simulink model "VehicleFollowing_R2019a"  (R2019a)
settings: Solver=VariableStepAuto  StartTime=0.0  StopTime=50  RelTol=1e-3
libraries: simulink x3, sim3dautolib x3, vrlib x2, sim3dlib x1, mpcadaslib x1, robotmobilelib x1
settings Model: Creator=Mustafa  LastModifiedBy=mustafa

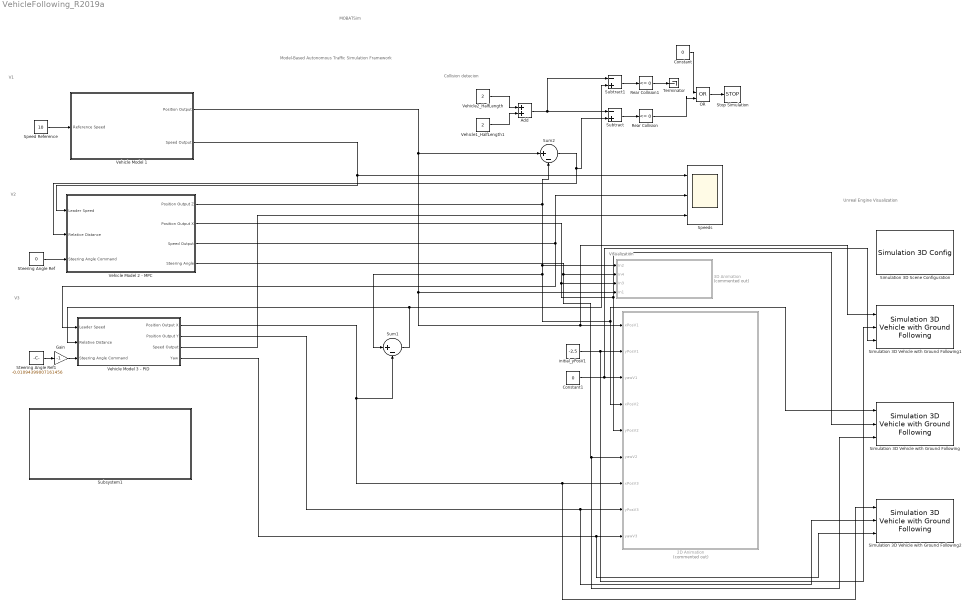
== system VehicleFollowing_R2019a ==
  note: Unreal Engine Visualization
  note: V1
  note: Visualization
  note: Collision detecion
  note: Model-Based Autonomous Traffic Simulation Framework
  note: MOBATSim
  note: V2
  note: V3
  2D Animation : Subsystem  Commented=on  TreatAsAtomicUnit=on  SystemSampleTime=0.02
  3D Animation : Subsystem  Commented=on
  Add : Sum
  Constant : Constant  Value=0
  Constant1 : Constant  Value=0
  Gain : Gain  Gain=-1
  OR : Logic  Operator=OR  IconShape=distinctive  AllPortsSameDT=off  OutDataTypeStr=boolean
  Rear Collision : simulink/Logic and Bit Operations/Compare To Constant  relop=<=  const=0  OutDataTypeStr=boolean
  Rear Collision1 : simulink/Logic and Bit Operations/Compare To Constant  relop=<=  const=0  OutDataTypeStr=boolean
  Simulation 3D Scene Configuration : sim3dlib/Simulation 3D Config  Priority=0  ProjectFormat=Default Scenes  SceneDesc=Straight road  ProjectName=VehicleSimulation.exe  vehTagList={'Scene Origin';'SimulinkVehicle1';'SimulinkVehicle2';'SimulinkVehicle3'}  vehTag=SimulinkVehicle3  OpVisEn=off  Ts=0.1  aMode=3
      settings: SourceProductBaseCode=DR,UV,VE
  Simulation 3D Vehicle with Ground Following : sim3dautolib/Simulation 3D Vehicle with Ground Following  Priority=-1  PassVehMesh=Small pickup truck  VehColor=Orange  InitialPos=[20, 0, 0]  InitialRot=[0, 0, 0]  ActorName=SimulinkVehicle1  SampleTime=0.1  ActorType=SimulinkVehicle  ID=1  aMode=3  ActorTag=SimulinkVehicle1  CoordinateScheme=ISO  TransformOutportEnabled=off
      settings: SourceProductBaseCode=DR,UV,VE
  Simulation 3D Vehicle with Ground Following1 : sim3dautolib/Simulation 3D Vehicle with Ground Following  Priority=-1  PassVehMesh=Muscle car  VehColor=Red  InitialPos=[40, 0, 0]  InitialRot=[0, 0, 0]  ActorName=SimulinkVehicle2  SampleTime=0.1  ActorType=SimulinkVehicle  ID=2  aMode=3  ActorTag=SimulinkVehicle2  CoordinateScheme=ISO  TransformOutportEnabled=off
      settings: SourceProductBaseCode=DR,UV,VE
  Simulation 3D Vehicle with Ground Following2 : sim3dautolib/Simulation 3D Vehicle with Ground Following  Priority=-1  PassVehMesh=Sedan  VehColor=Silver  InitialPos=[0, 0, 0]  InitialRot=[0, 0, 0]  ActorName=SimulinkVehicle3  SampleTime=0.1  ActorType=SimulinkVehicle  ID=3  aMode=3  ActorTag=SimulinkVehicle3  CoordinateScheme=ISO  TransformOutportEnabled=off
      settings: SourceProductBaseCode=DR,UV,VE
  Speed Reference : Constant  Value=10
  Speeds : Scope  NumInputPorts=3
  Steering Angle Ref : Constant  Value=0
  Steering Angle Ref1 : Constant  Value=-0.01094399007161456
  Stop Simulation : Stop
  Subsystem1 : Subsystem
  Subtract : Sum  Inputs=-+
  Subtract1 : Sum  Inputs=-+
  Sum1 : Sum  Inputs=|+-
  Sum2 : Sum  Inputs=|+-
  Terminator : Terminator
  Vehicle Model 1 : Subsystem  mask{Pos=40, Speed=20}
      mask prompts: Pos "Initial Position"; Speed "Initial Speed"
      mask TypeOptions Pos: Initial Position/Value
      mask TypeOptions Speed: Initial Speed/Value
  Vehicle Model 2 - MPC : Subsystem  mask{Pos=20, Speed=25}
      mask prompts: Pos "Initial Position"; Speed "Initial Speed"
      mask TypeOptions Pos: Initial Position Z/Value
      mask TypeOptions Speed: Initial Speed/Value
  Vehicle Model 3 - PID : Subsystem  mask{Pos=0, Speed=10}
      mask prompts: Pos "Initial Position"; Speed "Initial Speed"
      mask TypeOptions Pos: Initial Position X/Value
      mask TypeOptions Speed: Initial Speed/Value
  Vehicle1_HalfLength1 : Constant  Value=2
  Vehicle2_HalfLength : Constant  Value=2
  initial_yPosV1 : Constant  Value=-2.5
  wires:
  Vehicle Model 2 - MPC/1(Position Output Z) -> Sum1/1, 2D Animation/4(xPosV2), Simulation 3D Vehicle with Ground Following/1, 3D Animation/1(In2), Sum2/2
  Vehicle Model 2 - MPC/3(Speed Output) -> Vehicle Model 3 - PID/1(Leader Speed), Speeds/2
  Speed Reference/1 -> Vehicle Model 1/1(Reference Speed)
  Vehicle Model 1/1(Position Output) -> Sum2/1, Simulation 3D Vehicle with Ground Following1/1, 2D Animation/1(xPosV1), 3D Animation/4(In1)
  Sum2/1 -> Subtract/2, Vehicle Model 2 - MPC/2(Relative Distance)
  Vehicle Model 1/2(Speed Output) -> Vehicle Model 2 - MPC/1(Leader Speed), Speeds/1
  Steering Angle Ref/1 -> Vehicle Model 2 - MPC/3(Steering Angle Command)
  Vehicle Model 2 - MPC/2(Position Output X) -> 2D Animation/5(yPosV2), Simulation 3D Vehicle with Ground Following/2, 3D Animation/3(In3)
  Vehicle Model 2 - MPC/4(Steering Angle) -> Simulation 3D Vehicle with Ground Following/3, 2D Animation/6(yawV2), 3D Animation/2(In4)
  initial_yPosV1/1 -> Simulation 3D Vehicle with Ground Following1/2, 2D Animation/2(yPosV1)
  Constant1/1 -> Simulation 3D Vehicle with Ground Following1/3, 2D Animation/3(yawV1)
  Vehicle1_HalfLength1/1 -> Add/2
  Vehicle2_HalfLength/1 -> Add/1
  Add/1 -> Subtract1/1, Subtract/1
  Subtract/1 -> Rear Collision/1
  Vehicle Model 3 - PID/1(Position Output X) -> Simulation 3D Vehicle with Ground Following2/1, 2D Animation/7(xPosV3), Sum1/2
  Vehicle Model 3 - PID/2(Position Output Y) -> Simulation 3D Vehicle with Ground Following2/2, 2D Animation/8(yPosV3)
  Vehicle Model 3 - PID/3(Speed Output) -> Speeds/3
  Vehicle Model 3 - PID/4(Yaw) -> Simulation 3D Vehicle with Ground Following2/3, 2D Animation/9(yawV3)
  Sum1/1 -> Vehicle Model 3 - PID/2(Relative Distance), Subtract1/2
  OR/1 -> Stop Simulation/1
  Rear Collision/1 -> OR/2
  Subtract1/1 -> Rear Collision1/1
  Steering Angle Ref1/1 -> Gain/1
  Constant/1 -> OR/1
  Rear Collision1/1 -> Terminator/1
  Gain/1 -> Vehicle Model 3 - PID/3(Steering Angle Command)

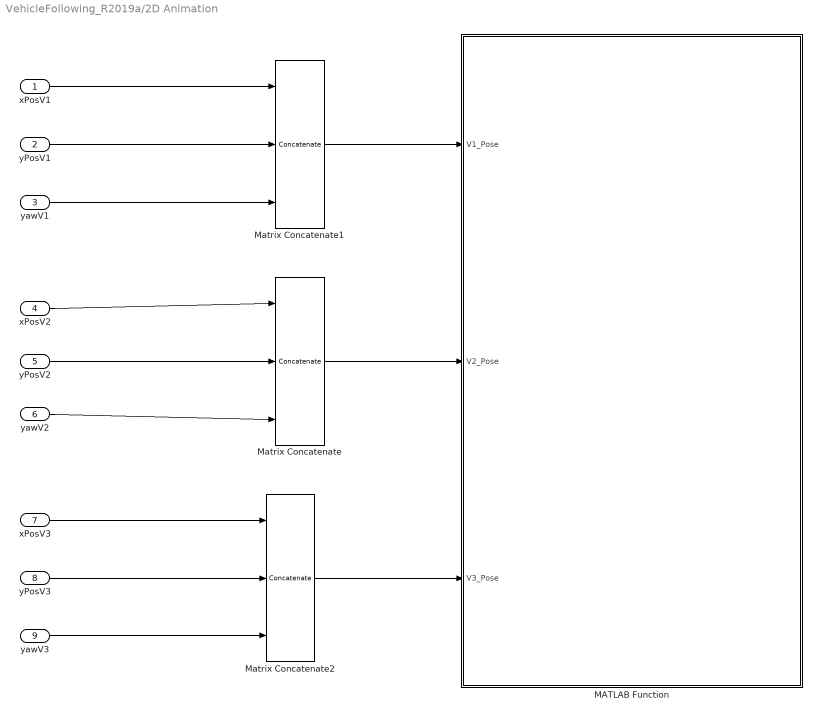
== system VehicleFollowing_R2019a/2D Animation ==
  xPosV1 : Inport
  yPosV1 : Inport  Port=2
  yawV1 : Inport  Port=3
  xPosV2 : Inport  Port=4
  yPosV2 : Inport  Port=5
  yawV2 : Inport  Port=6
  xPosV3 : Inport  Port=7
  yPosV3 : Inport  Port=8
  yawV3 : Inport  Port=9
  MATLAB Function : MATLAB Function  TreatAsAtomicUnit=on
      mask init:
      | close all;
      | figure('units','normalized','outerposition',[0 0 1 1]);
      | grid on
      | axis equal
      | hold on
  Matrix Concatenate : Concatenate  NumInputs=3  ConcatenateDimension=2
  Matrix Concatenate1 : Concatenate  NumInputs=3  ConcatenateDimension=2
  Matrix Concatenate2 : Concatenate  NumInputs=3  ConcatenateDimension=2
  wires:
  xPosV2/1 -> Matrix Concatenate/1
  Matrix Concatenate/1 -> MATLAB Function/2(V2_Pose)
  yPosV2/1 -> Matrix Concatenate/2
  yawV2/1 -> Matrix Concatenate/3
  Matrix Concatenate1/1 -> MATLAB Function/1(V1_Pose)
  xPosV1/1 -> Matrix Concatenate1/1
  yPosV1/1 -> Matrix Concatenate1/2
  yawV1/1 -> Matrix Concatenate1/3
  yPosV3/1 -> Matrix Concatenate2/2
  xPosV3/1 -> Matrix Concatenate2/1
  yawV3/1 -> Matrix Concatenate2/3
  Matrix Concatenate2/1 -> MATLAB Function/3(V3_Pose)

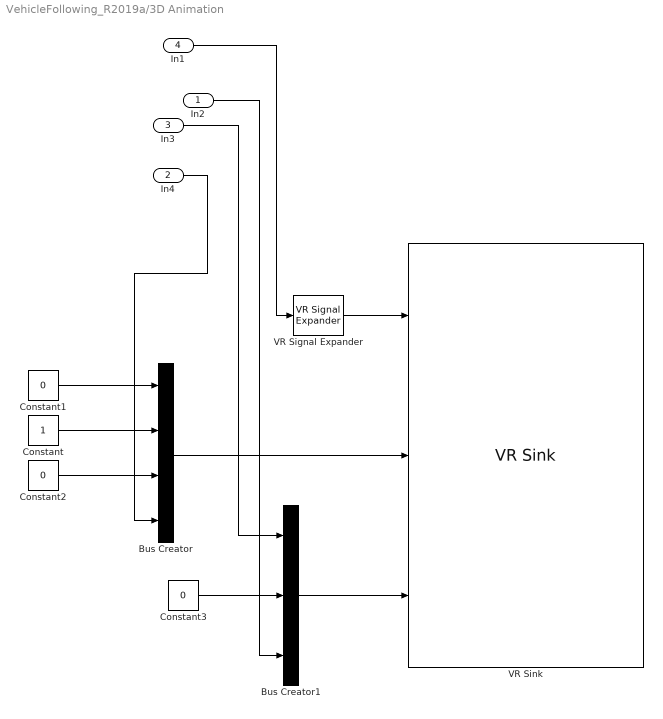
== system VehicleFollowing_R2019a/3D Animation ==
  In2 : Inport
  In4 : Inport  Port=2
  In3 : Inport  Port=3
  In1 : Inport  Port=4
  Bus Creator : BusCreator  Inputs=4
  Bus Creator1 : BusCreator  Inputs=3
  Constant : Constant
  Constant1 : Constant  Value=0
  Constant2 : Constant  Value=0
  Constant3 : Constant  Value=0
  VR Signal Expander : vrlib/VR Signal Expander  outwidth=3  outidx=[3]
  VR Sink : vrlib/VR Sink  InstantiateOnLoad=on  SampleTime=0.02  ViewEnable=on  RemoteChange=off  RemoteView=off  FieldsWritten=Car_Red.translation.3.1.1.double#Car_Blue.rotation.4.1.1.double#Car_Blue.translation.3.1.1.double  WorldFileName=PlatoonWorld.WRL  AutoView=off  VideoDimensions=[]  AllowVariableSize=off
  wires:
  Constant/1 -> Bus Creator/2
  Constant1/1 -> Bus Creator/1
  Bus Creator1/1 -> VR Sink/3
  In2/1 -> Bus Creator1/3
  Bus Creator/1 -> VR Sink/2
  In4/1 -> Bus Creator/4
  In1/1 -> VR Signal Expander/1
  Constant3/1 -> Bus Creator1/2
  Constant2/1 -> Bus Creator/3
  VR Signal Expander/1 -> VR Sink/1
  In3/1 -> Bus Creator1/1

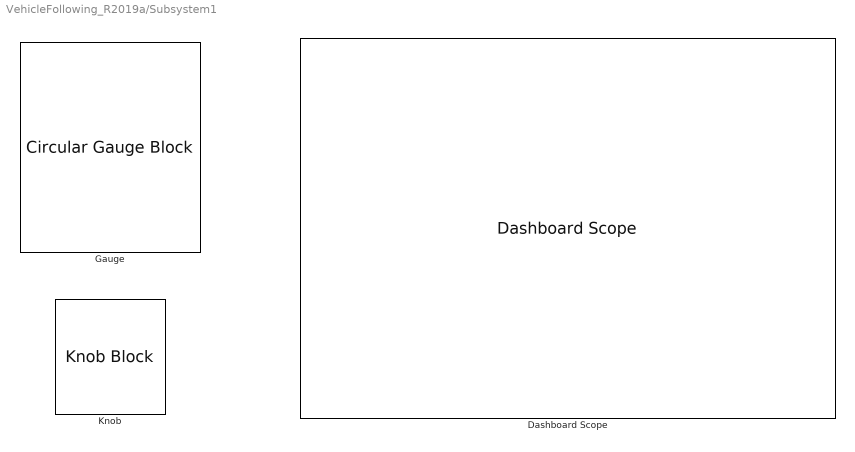
== system VehicleFollowing_R2019a/Subsystem1 ==
  Dashboard Scope : DashboardScope  WebBlockId=244
  Gauge : CircularGaugeBlock  WebBlockId=245
  Knob : KnobBlock  ScaleMin=-0.2  ScaleMax=0.2  WebBlockId=247

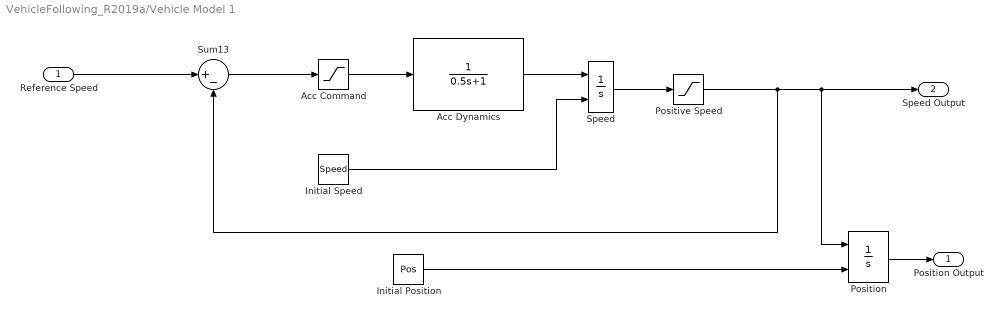
== system VehicleFollowing_R2019a/Vehicle Model 1 ==
  Reference Speed : Inport
  Acc Command : Saturate  UpperLimit=2  LowerLimit=-3
  Acc Dynamics : TransferFcn  Denominator=[0.5 1]
  Initial Position : Constant  Value=Pos
  Initial Speed : Constant  Value=Speed
  Position : Integrator  InitialConditionSource=external
  Positive Speed : Saturate  UpperLimit=inf  LowerLimit=0
  Speed : Integrator  InitialConditionSource=external
  Sum13 : Sum  Inputs=|+-
  Position Output : Outport  VectorParamsAs1DForOutWhenUnconnected=off
  Speed Output : Outport  Port=2  VectorParamsAs1DForOutWhenUnconnected=off
  wires:
  Speed/1 -> Positive Speed/1
  Positive Speed/1 -> Sum13/2, Speed Output/1, Position/1
  Initial Position/1 -> Position/2
  Sum13/1 -> Acc Command/1
  Reference Speed/1 -> Sum13/1
  Acc Command/1 -> Acc Dynamics/1
  Acc Dynamics/1 -> Speed/1
  Initial Speed/1 -> Speed/2
  Position/1 -> Position Output/1

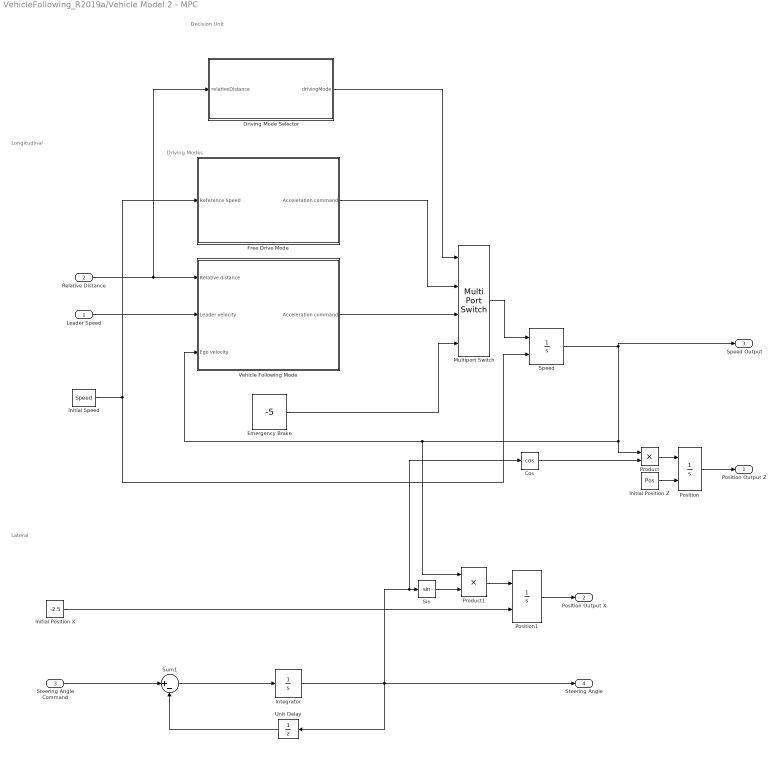
== system VehicleFollowing_R2019a/Vehicle Model 2 - MPC ==
  note: Decision Unit
  note: Driving Modes
  note: Longitudinal
  note: Lateral
  Leader Speed : Inport
  Relative Distance : Inport  Port=2
  Steering Angle Command : Inport  Port=3
  Cos : Trigonometry  Operator=cos
  Driving Mode Selector : Stateflow chart  TreatAsAtomicUnit=on
  Emergency Brake : Constant  Value=-5
  Free Drive Mode : Subsystem
  Initial Position X : Constant  Value=-2.5
  Initial Position Z : Constant  Value=Pos
  Initial Speed : Constant  Value=Speed
  Integrator : Integrator
  Multiport Switch : MultiPortSwitch
  Position : Integrator  InitialConditionSource=external
  Position1 : Integrator  InitialConditionSource=external
  Product : Product
  Product1 : Product
  Sin : Trigonometry
  Speed : Integrator  InitialConditionSource=external  LimitOutput=on  LowerSaturationLimit=0
  Sum1 : Sum  Inputs=|+-
  Unit Delay : UnitDelay  SampleTime=-1  HasFrameUpgradeWarning=on
  Vehicle Following Mode : Subsystem
  Position Output Z : Outport  VectorParamsAs1DForOutWhenUnconnected=off
  Position Output X : Outport  Port=2  VectorParamsAs1DForOutWhenUnconnected=off
  Speed Output : Outport  Port=3  VectorParamsAs1DForOutWhenUnconnected=off
  Steering Angle : Outport  Port=4  VectorParamsAs1DForOutWhenUnconnected=off
  wires:
  Position/1 -> Position Output Z/1
  Initial Speed/1 -> Free Drive Mode/1(Reference Speed), Speed/2
  Initial Position Z/1 -> Position/2
  Speed/1 -> Speed Output/1, Vehicle Following Mode/3(Ego velocity), Product1/1, Product/1
  Steering Angle Command/1 -> Sum1/1
  Sum1/1 -> Integrator/1
  Integrator/1 -> Unit Delay/1, Sin/1, Cos/1, Steering Angle/1
  Unit Delay/1 -> Sum1/2
  Initial Position X/1 -> Position1/2
  Cos/1 -> Product/2
  Product/1 -> Position/1
  Sin/1 -> Product1/2
  Product1/1 -> Position1/1
  Position1/1 -> Position Output X/1
  Relative Distance/1 -> Driving Mode Selector/1(relativeDistance), Vehicle Following Mode/1(Relative distance)
  Leader Speed/1 -> Vehicle Following Mode/2(Leader velocity)
  Vehicle Following Mode/1(Acceleration command) -> Multiport Switch/3
  Multiport Switch/1 -> Speed/1
  Free Drive Mode/1(Acceleration command) -> Multiport Switch/2
  Emergency Brake/1 -> Multiport Switch/4
  Driving Mode Selector/1(drivingMode) -> Multiport Switch/1

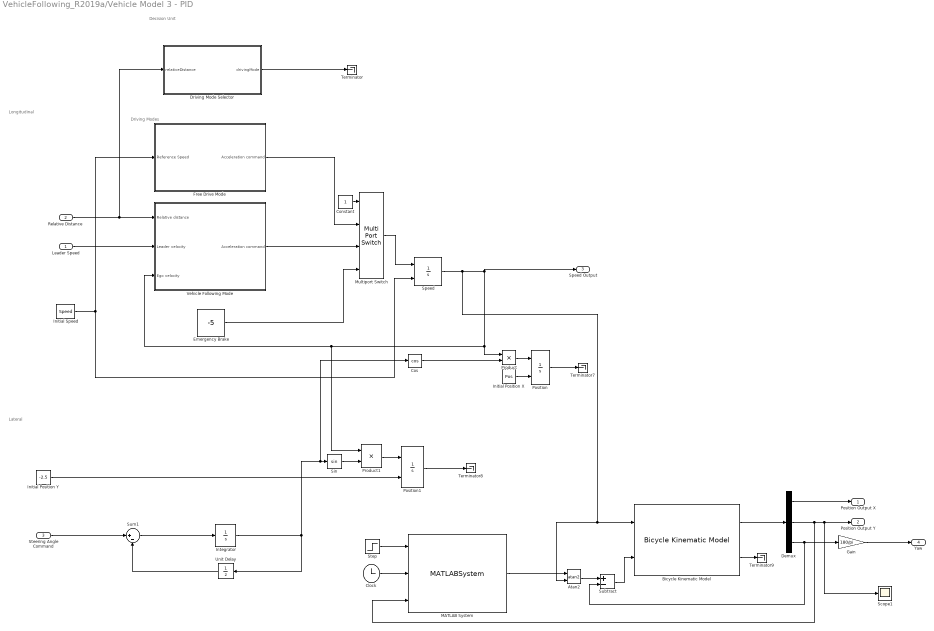
== system VehicleFollowing_R2019a/Vehicle Model 3 - PID ==
  note: Decision Unit
  note: Driving Modes
  note: Longitudinal
  note: Lateral
  Leader Speed : Inport
  Relative Distance : Inport  Port=2
  Steering Angle Command : Inport  Port=3
  Atan2 : Trigonometry  Operator=atan2
  Bicycle Kinematic Model : robotmobilelib/Bicycle Kinematic Model  VehicleInputs=Vehicle Speed & Steering Angle  WheelBase=3  VehicleSpeedRange=[0 12]  MaxSteeringAngle=pi/4  InitialState=[0; -3; 0]  SimulateUsing=Interpreted execution
      settings: SourceProductBaseCode=RO
  Clock : Clock
  Constant : Constant
  Cos : Trigonometry  Operator=cos
  Demux : Demux  Outputs=3
  Driving Mode Selector : Stateflow chart  TreatAsAtomicUnit=on
  Emergency Brake : Constant  Value=-5
  Free Drive Mode : Subsystem
  Gain : Gain  Gain=180/pi
  Initial Position X : Constant  Value=Pos
  Initial Position Y : Constant  Value=-2.5
  Initial Speed : Constant  Value=Speed
  Integrator : Integrator
  MATLAB System : MATLABSystem  System=LaneChanger  SimulateUsing=Interpreted execution
      mask Type: LaneChanger
      mask Display:
      | disp('LaneChanger');
      | port_label('input',1,'flag');
      | port_label('input',2,'clock');
      | port_label('input',3,'y');
      | port_label('output',1,'latSpeed');
  Multiport Switch : MultiPortSwitch
  Position : Integrator  InitialConditionSource=external
  Position1 : Integrator  InitialConditionSource=external
  Product : Product
  Product1 : Product
  Scope1 : Scope
  Sin : Trigonometry
  Speed : Integrator  InitialConditionSource=external  LimitOutput=on  UpperSaturationLimit=12  LowerSaturationLimit=0
  Step : Step  Time=3  SampleTime=0
  Subtract : Sum  Inputs=+-
  Sum1 : Sum  Inputs=|+-
  Terminator{,7..9} (4 alike) : Terminator
  Unit Delay : UnitDelay  SampleTime=-1  HasFrameUpgradeWarning=on
  Vehicle Following Mode : Subsystem
  Position Output X : Outport  VectorParamsAs1DForOutWhenUnconnected=off
  Position Output Y : Outport  Port=2  VectorParamsAs1DForOutWhenUnconnected=off
  Speed Output : Outport  Port=3  VectorParamsAs1DForOutWhenUnconnected=off
  Yaw : Outport  Port=4  VectorParamsAs1DForOutWhenUnconnected=off
  wires:
  Initial Speed/1 -> Free Drive Mode/1(Reference Speed), Speed/2
  Initial Position X/1 -> Position/2
  Speed/1 -> Atan2/2, Bicycle Kinematic Model/1, Speed Output/1, Vehicle Following Mode/3(Ego velocity), Product1/1, Product/1
  Sum1/1 -> Integrator/1
  Integrator/1 -> Unit Delay/1, Sin/1, Cos/1
  Unit Delay/1 -> Sum1/2
  Initial Position Y/1 -> Position1/2
  Cos/1 -> Product/2
  Product/1 -> Position/1
  Sin/1 -> Product1/2
  Product1/1 -> Position1/1
  Relative Distance/1 -> Driving Mode Selector/1(relativeDistance), Vehicle Following Mode/1(Relative distance)
  Leader Speed/1 -> Vehicle Following Mode/2(Leader velocity)
  Vehicle Following Mode/1(Acceleration command) -> Multiport Switch/3
  Multiport Switch/1 -> Speed/1
  Free Drive Mode/1(Acceleration command) -> Multiport Switch/2
  Emergency Brake/1 -> Multiport Switch/4
  Driving Mode Selector/1(drivingMode) -> Terminator/1
  Constant/1 -> Multiport Switch/1
  Position/1 -> Terminator7/1
  Position1/1 -> Terminator8/1
  Gain/1 -> Yaw/1
  Bicycle Kinematic Model/1 -> Demux/1
  Bicycle Kinematic Model/2 -> Terminator9/1
  Demux/3 -> Subtract/2, Gain/1
  Demux/2 -> MATLAB System/3, Scope1/1, Position Output Y/1
  Demux/1 -> Position Output X/1
  Steering Angle Command/1 -> Sum1/1
  Step/1 -> MATLAB System/1
  Clock/1 -> MATLAB System/2
  MATLAB System/1 -> Atan2/1
  Atan2/1 -> Subtract/1
  Subtract/1 -> Bicycle Kinematic Model/2

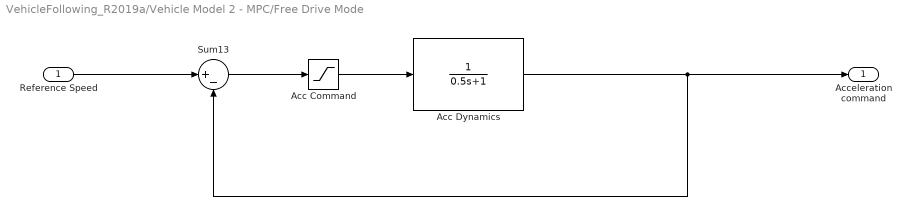
== system VehicleFollowing_R2019a/Vehicle Model 2 - MPC/Free Drive Mode ==
  Reference Speed : Inport
  Acc Command : Saturate  UpperLimit=2  LowerLimit=-3
  Acc Dynamics : TransferFcn  Denominator=[0.5 1]
  Sum13 : Sum  Inputs=|+-
  Acceleration command : Outport
  wires:
  Sum13/1 -> Acc Command/1
  Acc Dynamics/1 -> Acceleration command/1, Sum13/2
  Reference Speed/1 -> Sum13/1
  Acc Command/1 -> Acc Dynamics/1

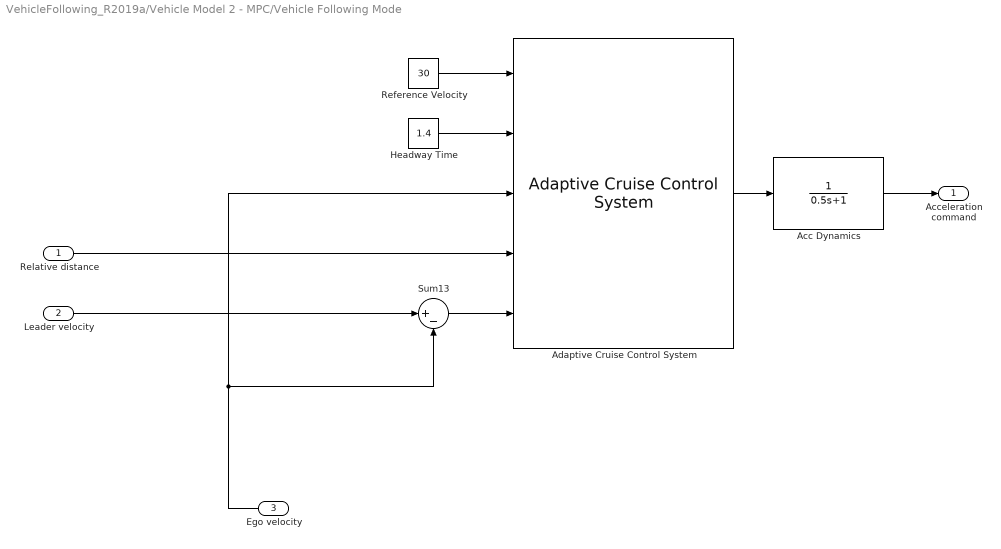
== system VehicleFollowing_R2019a/Vehicle Model 2 - MPC/Vehicle Following Mode ==
  Relative distance : Inport
  Leader velocity : Inport  Port=2
  Ego velocity : Inport  Port=3
  Acc Dynamics : TransferFcn  Denominator=[0.5 1]
  Adaptive Cruise Control System : mpcadaslib/Adaptive Cruise Control System  EgoModel=tf(1,[0.5,1,0])  InitialEgoVelocity=30  DefaultSpacing=10  MaxVelocity=50  MinAcceleration=-3  amin_ext=off  MaxAcceleration=2  amax_ext=off  Ts=0.5  PredictionHorizon=200  ControllerBehavior=0.590  suboptimal=off  maxiter=100  datatypeopt=double  optmode=off  trackmode=off
  Headway Time : Constant  Value=1.4
  Reference Velocity : Constant  Value=30
  Sum13 : Sum  Inputs=|+-
  Acceleration command : Outport
  wires:
  Leader velocity/1 -> Sum13/1
  Headway Time/1 -> Adaptive Cruise Control System/2
  Reference Velocity/1 -> Adaptive Cruise Control System/1
  Ego velocity/1 -> Adaptive Cruise Control System/3, Sum13/2
  Sum13/1 -> Adaptive Cruise Control System/5
  Relative distance/1 -> Adaptive Cruise Control System/4
  Adaptive Cruise Control System/1 -> Acc Dynamics/1
  Acc Dynamics/1 -> Acceleration command/1

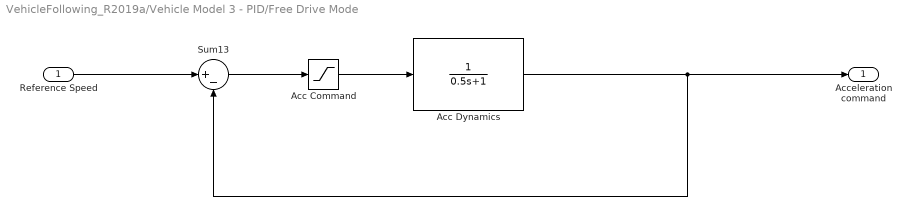
== system VehicleFollowing_R2019a/Vehicle Model 3 - PID/Free Drive Mode ==
  Reference Speed : Inport
  Acc Command : Saturate  UpperLimit=2  LowerLimit=-3
  Acc Dynamics : TransferFcn  Denominator=[0.5 1]
  Sum13 : Sum  Inputs=|+-
  Acceleration command : Outport
  wires:
  Sum13/1 -> Acc Command/1
  Acc Dynamics/1 -> Acceleration command/1, Sum13/2
  Reference Speed/1 -> Sum13/1
  Acc Command/1 -> Acc Dynamics/1

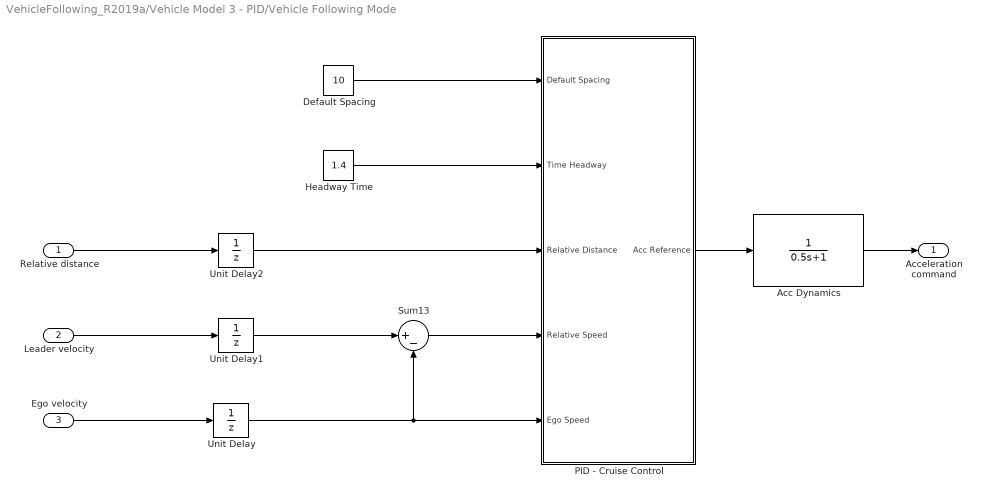
== system VehicleFollowing_R2019a/Vehicle Model 3 - PID/Vehicle Following Mode ==
  Relative distance : Inport
  Leader velocity : Inport  Port=2
  Ego velocity : Inport  Port=3
  Acc Dynamics : TransferFcn  Denominator=[0.5 1]
  Default Spacing : Constant  Value=10
  Headway Time : Constant  Value=1.4
  PID - Cruise Control : Subsystem
  Sum13 : Sum  Inputs=|+-
  Unit Delay : UnitDelay  SampleTime=-1  HasFrameUpgradeWarning=on
  Unit Delay1 : UnitDelay  SampleTime=-1  HasFrameUpgradeWarning=on
  Unit Delay2 : UnitDelay  SampleTime=-1  HasFrameUpgradeWarning=on
  Acceleration command : Outport
  wires:
  Leader velocity/1 -> Unit Delay1/1
  Headway Time/1 -> PID - Cruise Control/2(Time Headway)
  Ego velocity/1 -> Unit Delay/1
  Sum13/1 -> PID - Cruise Control/4(Relative Speed)
  Relative distance/1 -> Unit Delay2/1
  PID - Cruise Control/1(Acc Reference) -> Acc Dynamics/1
  Acc Dynamics/1 -> Acceleration command/1
  Default Spacing/1 -> PID - Cruise Control/1(Default Spacing)
  Unit Delay/1 -> Sum13/2, PID - Cruise Control/5(Ego Speed)
  Unit Delay1/1 -> Sum13/1
  Unit Delay2/1 -> PID - Cruise Control/3(Relative Distance)

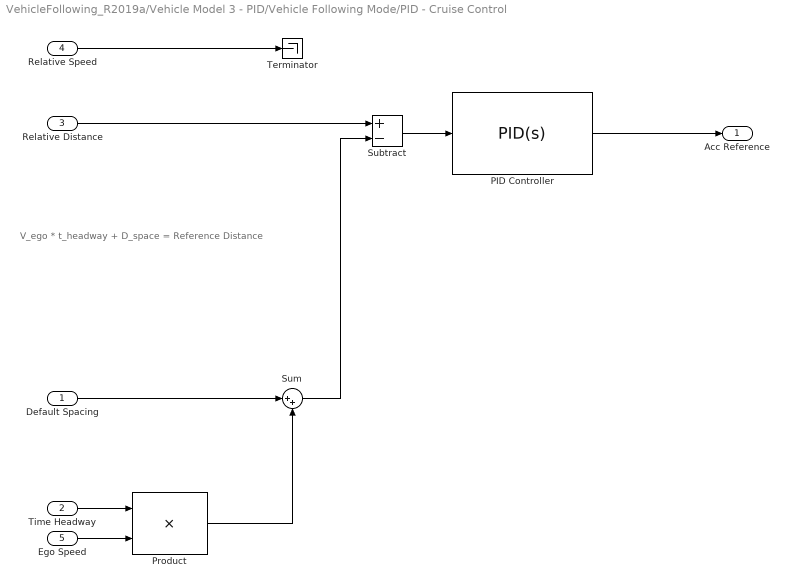
== system VehicleFollowing_R2019a/Vehicle Model 3 - PID/Vehicle Following Mode/PID - Cruise Control ==
  note: V_ego * t_headway + D_space = Reference Distance
  Default Spacing : Inport
  Time Headway : Inport  Port=2
  Relative Distance : Inport  Port=3
  Relative Speed : Inport  Port=4
  Ego Speed : Inport  Port=5
  PID Controller : simulink/Continuous/PID Controller  Controller=PID  Form=Parallel  TimeDomain=Continuous-time  SampleTime=-1  IntegratorMethod=Forward Euler  FilterMethod=Forward Euler  ControllerParametersSource=internal  P=2  I=0.04  D=2.1  UseFilter=on  N=230  TunerSelectOption=Transfer Function Based (PID Tuner App)  InitialConditionSource=internal  InitialConditionForIntegrator=0  InitialConditionForFilter=0  DifferentiatorICPrevScaledInput=0  ExternalReset=none  TrackingMode=off  Kt=1  LimitOutput=on  UpperSaturationLimit=2  LowerSaturationLimit=-3  LinearizeAsGain=on  AntiWindupMode=clamping  Kb=1  POutMin=[]  POutMax=[]  IOutMin=[]  IOutMax=[]  DOutMin=[]  DOutMax=[]  NOutMin=[]  NOutMax=[]  SumOutMin=[]  SumOutMax=[]  SaturationOutMin=[]  SaturationOutMax=[]  PParamMin=[]  PParamMax=[]  IParamMin=[]  IParamMax=[]  DParamMin=[]  DParamMax=[]  NParamMin=[]  NParamMax=[]  KbParamMin=[]  KbParamMax=[]  KtParamMin=[]  KtParamMax=[]  KbOutMin=[]  KbOutMax=[]  KtOutMin=[]  KtOutMax=[]  IntegratorOutMin=[]  IntegratorOutMax=[]  FilterOutMin=[]  FilterOutMax=[]  SumI1OutMin=[]  SumI1OutMax=[]  SumI2OutMin=[]  SumI2OutMax=[]  SumI3OutMin=[]  SumI3OutMax=[]  SumI4OutMin=[]  SumI4OutMax=[]  SumDOutMin=[]  SumDOutMax=[]  DifferentiatorOutMin=[]  DifferentiatorOutMax=[]  FilterDiffOutCoefMin=[]  FilterDiffOutCoefMax=[]  ReciprocalOutMin=[]  ReciprocalOutMax=[]  SumDenOutMin=[]  SumDenOutMax=[]  SumNumOutMin=[]  SumNumOutMax=[]  DivideOutMin=[]  DivideOutMax=[]  IntegratorContinuousStateAttributes=''  IntegratorStateMustResolveToSignalObject=off  IntegratorRTWStateStorageClass=Auto  FilterContinuousStateAttributes=''  FilterStateMustResolveToSignalObject=off  FilterRTWStateStorageClass=Auto  ParallelPVariant=InternalParameters  IdealPVariant=Disabled  IVariant=InternalParameters  DVariant=InternalParameters  IntegratorVariant=Continuous  SatVariant=Enabled  AWVariant=ContClampingParallel  PCopyVariant=Disabled  TRVariant=Disabled  FdbkBlocksVariant=Forward  IdealPFdbkVariant=Disabled  SatFdbkVariant=Disabled  DerivativeFilterVariant=ContFilter  NVariant=InternalParameters  NCopyVariant=Disabled  FilterICVariant=InternalICsFilter  IntegratorICVariant=InternalICs  ExternalResetVariant=Disabled  TRSumVariant=Passthrough  SumFdbkVariant=Disabled  SumVariant=Sum_PID
  Product : Product
  Subtract : Sum  Inputs=+-
  Sum : Sum  Inputs=|++
  Terminator : Terminator
  Acc Reference : Outport
  wires:
  Ego Speed/1 -> Product/2
  Time Headway/1 -> Product/1
  Default Spacing/1 -> Sum/1
  Product/1 -> Sum/2
  Sum/1 -> Subtract/2
  Relative Distance/1 -> Subtract/1
  Subtract/1 -> PID Controller/1
  PID Controller/1 -> Acc Reference/1
  Relative Speed/1 -> Terminator/1

== stateflow chart VehicleFollowing_R2019a/Vehicle Model 3 - PID/Driving Mode Selector ==
  state VehicleFollowing
    entry:
    drivingMode=2;
  state FreeDrive
    entry:
    drivingMode =1;
  state EmergecyBrake
    entry:
    drivingMode=3;
  (default) -> FreeDrive
  VehicleFollowing -> FreeDrive [order 1] : [relativeDistance >50]
  FreeDrive -> VehicleFollowing [order 1] : [relativeDistance <=40]
  FreeDrive -> EmergecyBrake [order 2] : [relativeDistance <=10]
  VehicleFollowing -> EmergecyBrake [order 2] : [relativeDistance <=10]
  EmergecyBrake -> VehicleFollowing : [relativeDistance>15]
  data: relativeDistance input; drivingMode output

== matlab function VehicleFollowing_R2019a/2D Animation/MATLAB Function ==
  data: V1_Pose input; V2_Pose input; V3_Pose input
function plotVehicle(V1_Pose, V2_Pose, V3_Pose)
%% Clear previous Vehicle
cla;

%% Vehicle 1 - Pose
x1 = V1_Pose(1);
y1 = V1_Pose(2);
yaw1 = V1_Pose(3);

centerP = [x1;y1];

V1_HalfLength = 2; % Length = 4m
V1_HalfWidth = 1; % Width = 2m

% Creating a rectangle
p1 = [V1_HalfLength; V1_HalfWidth];
p2 = [V1_HalfLength; -V1_HalfWidth];
p3 = [-V1_HalfLength; -V1_HalfWidth];
p4 = [-V1_HalfLength; V1_HalfWidth];

% Rotation Matrix
Rmatrix = [cos(yaw1) -sin(yaw1); sin(yaw1) cos(yaw1)];

% Rotated Points
p1r = centerP + Rmatrix*p1;
p2r = centerP + Rmatrix*p2;
p3r = centerP + Rmatrix*p3;
p4r = centerP + Rmatrix*p4;

% Connecting points
Hitbox_V1 = [p1r p2r p3r p4r p1r];

cornersV1_x = transpose(Hitbox_V1(1,:));
cornersV1_y = transpose(Hitbox_V1(2,:));

%% Vehicle 2 - Pose
x2 = V2_Pose(1);
y2 = V2_Pose(2);
yaw2 = V2_Pose(3);

centerP = [x2;y2];

V2_HalfLength = 2; % Length = 4m
V2_HalfWidth = 1; % Width = 2m

% Creating a rectangle
p1 = [V2_HalfLength; V2_HalfWidth];
p2 = [V2_HalfLength; -V2_HalfWidth];
p3 = [-V2_HalfLength; -V2_HalfWidth];
p4 = [-V2_HalfLength; V2_HalfWidth];

% Rotation Matrix

Rmatrix = [cos(yaw2) -sin(yaw2); sin(yaw2) cos(yaw2)];

% Rotated Points
p1r = centerP + Rmatrix*p1;
p2r = centerP + Rmatrix*p2;
p3r = centerP + Rmatrix*p3;
p4r = centerP + Rmatrix*p4;

% Connecting points
Hitbox_V2 = [p1r p2r p3r p4r p1r];

cornersV2_x = transpose(Hitbox_V2(1,:));
cornersV2_y = transpose(Hitbox_V2(2,:));

%% Vehicle 3 - Pose
x3 = V3_Pose(1);
y3 = V3_Pose(2);
yaw3 = V3_Pose(3);

centerP = [x3;y3];

V3_HalfLength = 2; % Length = 4m
V3_HalfWidth = 1; % Width = 2m

% Creating a rectangle
p1 = [V3_HalfLength; V3_HalfWidth];
p2 = [V3_HalfLength; -V3_HalfWidth];
p3 = [-V3_HalfLength; -V3_HalfWidth];
p4 = [-V3_HalfLength; V3_HalfWidth];

% Rotation Matrix
Rmatrix = [cos(yaw3) -sin(yaw3); sin(yaw3) cos(yaw3)];

% Rotated Points
p1r = centerP + Rmatrix*p1;
p2r = centerP + Rmatrix*p2;
p3r = centerP + Rmatrix*p3;
p4r = centerP + Rmatrix*p4;

% Connecting points
Hitbox_V3 = [p1r p2r p3r p4r p1r];

cornersV3_x = transpose(Hitbox_V3(1,:));
cornersV3_y = transpose(Hitbox_V3(2,:));

%% Plot Vehicles and the road
plot(cornersV1_x,cornersV1_y,'g'); %Vehicle 1 rectangle
plot(x1,y1,'*'); %Vehicle 1 center

plot(cornersV2_x,cornersV2_y,'r'); %Vehicle 2 rectangle
plot(x2,y2,'o'); %Vehicle 2 center

plot(cornersV3_x,cornersV3_y,'b'); %Vehicle 3 rectangle
plot(x3,y3,'x'); %Vehicle 3 center

upperLine = plot([0 1000], [5 5], 'Color', 'blue');
midLine = plot([0 1000], [0 0],'--', 'Color', 'blue');
lowerLine = plot([0 1000], [-5 -5], 'Color', 'blue');



% Adjust Axis
axis([x3-40 x3+40 y3-20 y3+20]); % Camera following V3 as ego vehicle

== stateflow chart VehicleFollowing_R2019a/Vehicle Model 2 - MPC/Driving Mode Selector ==
  state VehicleFollowing
    entry:
    drivingMode=2;
  state FreeDrive
    entry:
    drivingMode =1;
  state EmergecyBrake
    entry:
    drivingMode=3;
  (default) -> FreeDrive
  VehicleFollowing -> FreeDrive [order 1] : [relativeDistance >50]
  FreeDrive -> VehicleFollowing [order 1] : [relativeDistance <=40]
  FreeDrive -> EmergecyBrake [order 2] : [relativeDistance <=10]
  VehicleFollowing -> EmergecyBrake [order 2] : [relativeDistance <=10]
  EmergecyBrake -> VehicleFollowing : [relativeDistance>15]
  data: relativeDistance input; drivingMode output
